simulink model "adip_lqr2_sim"  (R2013a)
settings: Solver=ode1  StartTime=0.0  StopTime=3  FixedStep=0.001  RelTol=1e-3
values from neighbouring files (symbols this model uses):
  alpha2 = (Jp2 + mp2*lp2^2)/(mp2*lp2)    (= 0.353529459569)    [p1c511_ex4_cdip.m]
  dtheta1_0 = 0    [p1c523_ex8_adip_lqr.m]    (also in p1c523_ex8_adip_lqr_plot.m)
  dtheta2_0 = 0    [p1c523_ex8_adip_lqr.m]    (also in p1c523_ex8_adip_lqr_plot.m)
  K = [ k1  k2 ]    [p1c522_ex6.m]    (also in p1c522_ex7_adip_place.m = - place(A,B,s); p1c523_ex8_adip_lqr.m = - lqr(A,B,Q,R); p1c523_ex8_adip_lqr_plot.m = - lqr(A,B,Q,R))
  theta1_0 = 0    [p1c523_ex8_adip_lqr.m]    (also in p1c523_ex8_adip_lqr_plot.m)
  theta1e = pi/4    (= 0.785398163397)    [p1c522_ex7_adip_place.m]    (also in p1c523_ex8_adip_lqr.m; p1c523_ex8_adip_lqr_plot.m)
  theta2_0 = 0    [p1c523_ex8_adip_lqr.m]    (also in p1c523_ex8_adip_lqr_plot.m)
undefined symbols (not defined in the file or in its folder): a1, alpha3, alpha5, b1, mu2
settings Model: Creator=kawata  LastModifiedBy=kawata
settings DataIOCC: LimitDataPoints=off  SignalLoggingSaveFormat=ModelDataLogs
settings OptimizationCC: ExpressionDepthLimit=2147483647
settings DebuggingCC: FcnCallInpInsideContextMsg=UseLocalSettings
settings GRTTargetCC: CombineOutputUpdateFcns=off  GRTInterface=on

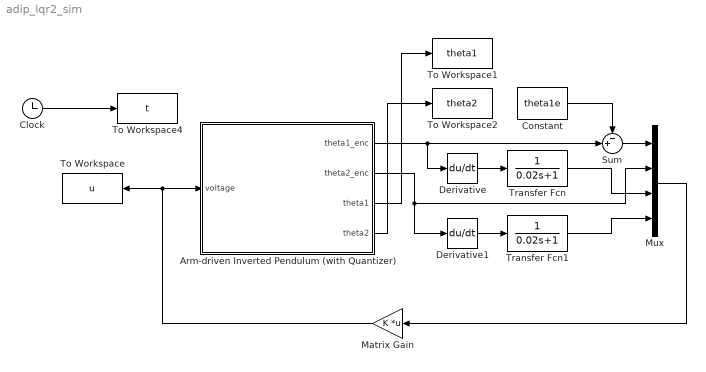
== system adip_lqr2_sim ==
  Arm-driven Inverted Pendulum (with Quantizer) : Subsystem
      mask Display: image(imread('adip_photo.jpg'),'center')
  Clock : Clock
  Constant : Constant  Value=theta1e
  Derivative : Derivative
  Derivative1 : Derivative
  Matrix Gain : Gain  Gain=K  Multiplication=Matrix(K*u)  SaturateOnIntegerOverflow=on  OutDataTypeStr=Inherit: Same as input  ParamDataTypeStr=Inherit: Same as input
  Mux : Mux
  Sum : Sum  Inputs=-+|
  To Workspace : ToWorkspace  VariableName=u  SampleTime=-1
  To Workspace1 : ToWorkspace  VariableName=theta1  SampleTime=-1
  To Workspace2 : ToWorkspace  VariableName=theta2  SampleTime=-1
  To Workspace4 : ToWorkspace  VariableName=t  SampleTime=-1
  Transfer Fcn : TransferFcn  Denominator=[0.02 1]
  Transfer Fcn1 : TransferFcn  Denominator=[0.02 1]
  wires:
  Arm-driven Inverted Pendulum (with Quantizer)/1(theta1_enc) -> Sum/2, Derivative/1
  Arm-driven Inverted Pendulum (with Quantizer)/2(theta2_enc) -> Derivative1/1, Mux/2
  Derivative/1 -> Transfer Fcn/1
  Derivative1/1 -> Transfer Fcn1/1
  Mux/1 -> Matrix Gain/1
  Transfer Fcn/1 -> Mux/3
  Transfer Fcn1/1 -> Mux/4
  Clock/1 -> To Workspace4/1
  Constant/1 -> Sum/1
  Sum/1 -> Mux/1
  Matrix Gain/1 -> Arm-driven Inverted Pendulum (with Quantizer)/1(voltage), To Workspace/1
  Arm-driven Inverted Pendulum (with Quantizer)/3(theta1) -> To Workspace1/1
  Arm-driven Inverted Pendulum (with Quantizer)/4(theta2) -> To Workspace2/1

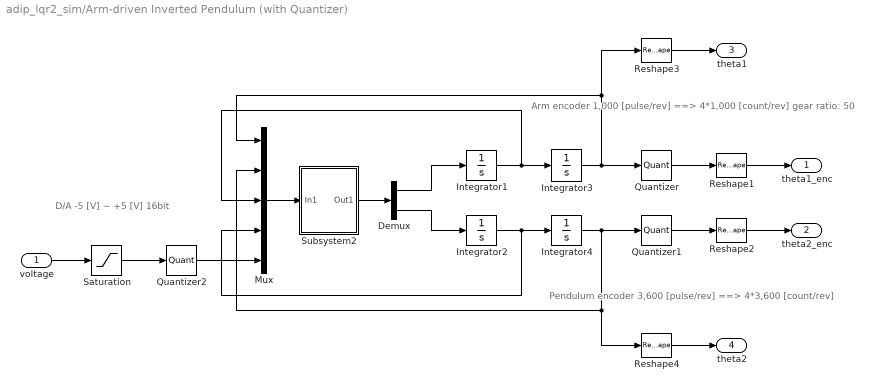
== system adip_lqr2_sim/Arm-driven Inverted Pendulum (with Quantizer) ==
  note: Pendulum encoder
      |   3,600 [pulse/rev]  ==> 4*3,600 [count/rev]
  note: Arm encoder
      |   1,000 [pulse/rev]  ==> 4*1,000 [count/rev]
      |   gear ratio: 50
  note: D/A
      |   -5 [V] ~ +5 [V]
      |  16bit
  voltage : Inport
  Demux : Demux  Outputs=2
  Integrator1 : Integrator  InitialCondition=dtheta1_0
  Integrator2 : Integrator  InitialCondition=dtheta2_0
  Integrator3 : Integrator  InitialCondition=theta1_0
  Integrator4 : Integrator  InitialCondition=theta2_0
  Mux : Mux  Inputs=5
  Quantizer : Quantizer  QuantizationInterval=2*pi/(4*1000*50)
  Quantizer1 : Quantizer  QuantizationInterval=2*pi/(4*3600)
  Quantizer2 : Quantizer  QuantizationInterval=10/2^(16)
  Reshape{1..4} (4 alike) : Reshape
  Saturation : Saturate  UpperLimit=5  LowerLimit=-5
  Subsystem2 : Subsystem
  theta1_enc : Outport
  theta2_enc : Outport  Port=2
  theta1 : Outport  Port=3
  theta2 : Outport  Port=4
  wires:
  Reshape4/1 -> theta2/1
  Reshape3/1 -> theta1/1
  Subsystem2/1(Out1) -> Demux/1
  Mux/1 -> Subsystem2/1(In1)
  Demux/1 -> Integrator1/1
  Demux/2 -> Integrator2/1
  Integrator1/1 -> Integrator3/1, Mux/3
  Integrator2/1 -> Integrator4/1, Mux/4
  Integrator3/1 -> Reshape3/1, Mux/1, Quantizer/1
  Integrator4/1 -> Reshape4/1, Mux/2, Quantizer1/1
  Quantizer2/1 -> Mux/5
  Reshape2/1 -> theta2_enc/1
  Reshape1/1 -> theta1_enc/1
  voltage/1 -> Saturation/1
  Quantizer/1 -> Reshape1/1
  Quantizer1/1 -> Reshape2/1
  Saturation/1 -> Quantizer2/1

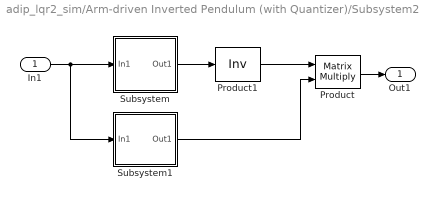
== system adip_lqr2_sim/Arm-driven Inverted Pendulum (with Quantizer)/Subsystem2 ==
  In1 : Inport
  Product : Product  Multiplication=Matrix(*)  SaturateOnIntegerOverflow=on  InputSameDT=on  OutDataTypeStr=Inherit: Same as first input
  Product1 : Product  Inputs=/  Multiplication=Matrix(*)  SaturateOnIntegerOverflow=on  InputSameDT=on  OutDataTypeStr=Inherit: Same as first input
  Subsystem : Subsystem
  Subsystem1 : Subsystem
  Out1 : Outport
  wires:
  Subsystem/1(Out1) -> Product1/1
  Product1/1 -> Product/1
  Subsystem1/1(Out1) -> Product/2
  In1/1 -> Subsystem/1(In1), Subsystem1/1(In1)
  Product/1 -> Out1/1

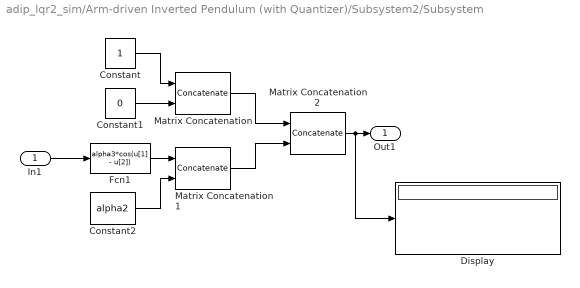
== system adip_lqr2_sim/Arm-driven Inverted Pendulum (with Quantizer)/Subsystem2/Subsystem ==
  In1 : Inport
  Constant : Constant
  Constant1 : Constant  Value=0
  Constant2 : Constant  Value=alpha2
  Display : Display
  Fcn1 : Fcn  Expr=alpha3*cos(u[1] - u[2])
  Matrix Concatenation : Concatenate  Mode=Multidimensional array  ConcatenateDimension=2
  Matrix Concatenation1 : Concatenate  Mode=Multidimensional array  ConcatenateDimension=2
  Matrix Concatenation2 : Concatenate  Mode=Multidimensional array
  Out1 : Outport
  wires:
  Constant2/1 -> Matrix Concatenation1/2
  Fcn1/1 -> Matrix Concatenation1/1
  In1/1 -> Fcn1/1
  Matrix Concatenation/1 -> Matrix Concatenation2/1
  Matrix Concatenation1/1 -> Matrix Concatenation2/2
  Matrix Concatenation2/1 -> Display/1, Out1/1
  Constant/1 -> Matrix Concatenation/1
  Constant1/1 -> Matrix Concatenation/2

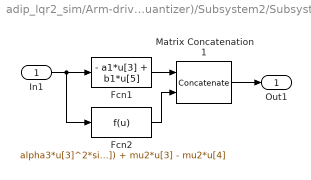
== system adip_lqr2_sim/Arm-driven Inverted Pendulum (with Quantizer)/Subsystem2/Subsystem1 ==
  In1 : Inport
  Fcn1 : Fcn  Expr=- a1*u[3] + b1*u[5]
  Fcn2 : Fcn  Expr=alpha3*u[3]^2*sin(u[1] - u[2]) + alpha5*sin(u[2]) + mu2*u[3] - mu2*u[4]
  Matrix Concatenation1 : Concatenate  Mode=Multidimensional array
  Out1 : Outport
  wires:
  Fcn2/1 -> Matrix Concatenation1/2
  Fcn1/1 -> Matrix Concatenation1/1
  In1/1 -> Fcn2/1, Fcn1/1
  Matrix Concatenation1/1 -> Out1/1
